simulink model "ssp_system"  (Simulink 6.5)
settings: Solver=ode45  StartTime=0.0  StopTime=10.0  RelTol=1e-3
libraries: nort_sysgenlib x7, xbsIndex_r4 x1
settings Model: Creator=nort  LastModifiedBy=nort

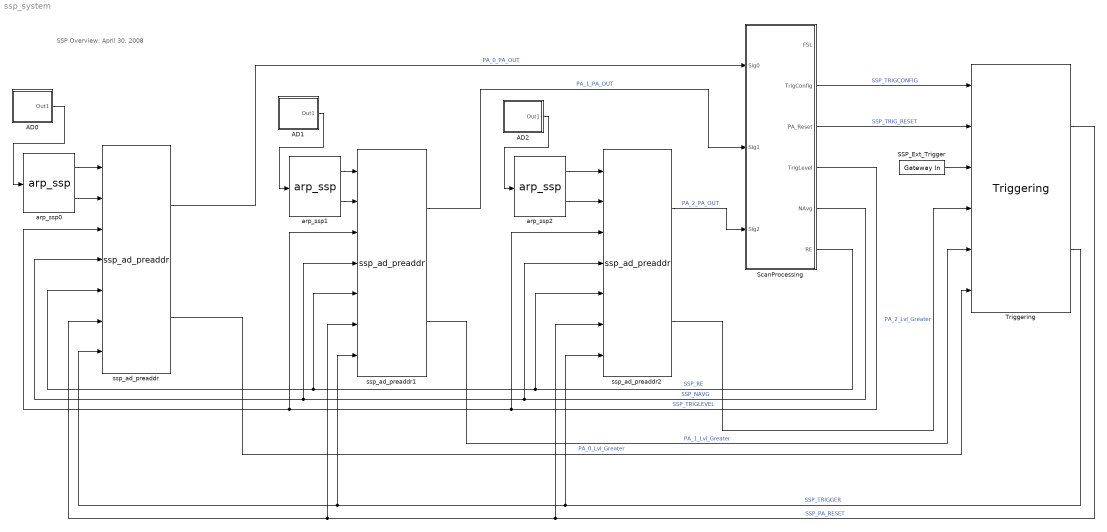
== system ssp_system ==
  note: SSP Overview: April 30, 2008
  AD0 : Subsystem
  AD1 : Subsystem
  AD2 : Subsystem
  SSP_Ext_Trigger : xbsIndex_r4/Gateway In  arith_type="Signed  (2's comp)"  n_bits=16  bin_pt=14  quantization="Round  (unbiased: +/- Inf)"  overflow=Saturate  period=1  dbl_ovrd=off  timing_constraint=None  locs_specified=off  LOCs={}  block_type=gatewayin
      settings: infoedit="Gateway in block.  Converts inputs of type Simulink integer, double and fixed point to  Xilinx fixed point type.<P><P>Hardware notes:  In hardware these blocks become top level input ports."  block_version=9.2.01
  ScanProcessing : Subsystem
  Triggering : nort_sysgenlib/Triggering  SystemSampleTime=-1
  arp_ssp0 : nort_sysgenlib/arp_ssp  SystemSampleTime=-1
  arp_ssp1 : nort_sysgenlib/arp_ssp  SystemSampleTime=-1
  arp_ssp2 : nort_sysgenlib/arp_ssp  SystemSampleTime=-1
  ssp_ad_preaddr : nort_sysgenlib/ssp_ad_preaddr  SystemSampleTime=-1
  ssp_ad_preaddr1 : nort_sysgenlib/ssp_ad_preaddr  SystemSampleTime=-1
  ssp_ad_preaddr2 : nort_sysgenlib/ssp_ad_preaddr  SystemSampleTime=-1
  wires:
  Triggering/2 -> ssp_ad_preaddr/7, ssp_ad_preaddr1/7, ssp_ad_preaddr2/7  "SSP_TRIGGER"
  arp_ssp0/1 -> ssp_ad_preaddr/1
  arp_ssp1/1 -> ssp_ad_preaddr1/1
  ScanProcessing/2(TrigConfig) -> Triggering/1  "SSP_TRIGCONFIG"
  ScanProcessing/5(NAvg) -> ssp_ad_preaddr/4, ssp_ad_preaddr1/4, ssp_ad_preaddr2/4  "SSP_NAVG"
  ScanProcessing/4(TrigLevel) -> ssp_ad_preaddr/3, ssp_ad_preaddr1/3, ssp_ad_preaddr2/3  "SSP_TRIGLEVEL"
  Triggering/1 -> ssp_ad_preaddr/6, ssp_ad_preaddr1/6, ssp_ad_preaddr2/6  "SSP_PA_RESET"
  ScanProcessing/3(PA_Reset) -> Triggering/2  "SSP_TRIG_RESET"
  ScanProcessing/6(RE) -> ssp_ad_preaddr/5, ssp_ad_preaddr1/5, ssp_ad_preaddr2/5  "SSP_RE"
  ssp_ad_preaddr2/1 -> ScanProcessing/3(Sig2)  "PA_2_PA_OUT"
  ssp_ad_preaddr1/1 -> ScanProcessing/2(Sig1)  "PA_1_PA_OUT"
  ssp_ad_preaddr/1 -> ScanProcessing/1(Sig0)  "PA_0_PA_OUT"
  ssp_ad_preaddr/2 -> Triggering/6  "PA_0_Lvl_Greater"
  ssp_ad_preaddr1/2 -> Triggering/5  "PA_1_Lvl_Greater"
  ssp_ad_preaddr2/2 -> Triggering/4  "PA_2_Lvl_Greater"
  SSP_Ext_Trigger/1 -> Triggering/3
  AD0/1(Out1) -> arp_ssp0/1
  AD1/1(Out1) -> arp_ssp1/1
  arp_ssp0/2 -> ssp_ad_preaddr/2
  arp_ssp1/2 -> ssp_ad_preaddr1/2
  arp_ssp2/1 -> ssp_ad_preaddr2/1
  arp_ssp2/2 -> ssp_ad_preaddr2/2
  AD2/1(Out1) -> arp_ssp2/1

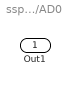
== system ssp_system/AD0 ==
  Out1 : Outport

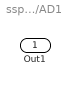
== system ssp_system/AD1 ==
  Out1 : Outport

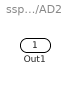
== system ssp_system/AD2 ==
  Out1 : Outport

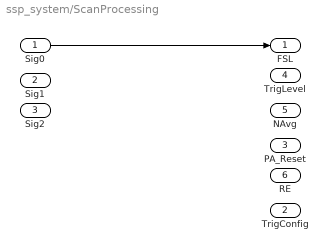
== system ssp_system/ScanProcessing ==
  Sig0 : Inport
  Sig1 : Inport  Port=2
  Sig2 : Inport  Port=3
  FSL : Outport
  TrigConfig : Outport  Port=2
  PA_Reset : Outport  Port=3
  TrigLevel : Outport  Port=4
  NAvg : Outport  Port=5
  RE : Outport  Port=6
  wires:
  Sig0/1 -> FSL/1
